simulink subsystem "DiscreteTimeController"  (R2020b)
settings: Solver=VariableStepAuto  StartTime=0.0  StopTime=10.0  RelTol=1e-3
model mask{Ts=-1, forward_action_enabled=0, use_lambda_const=on, lambdaT_const=0, use_max_analytic_lambda=on, rmse_noise_level=0, l_fcn_disabled=on, val_min=[], rmse_noise_slope_max=[], rmse_noise_min=[]}
settings Model: Creator=marco  LastModifiedBy=marco

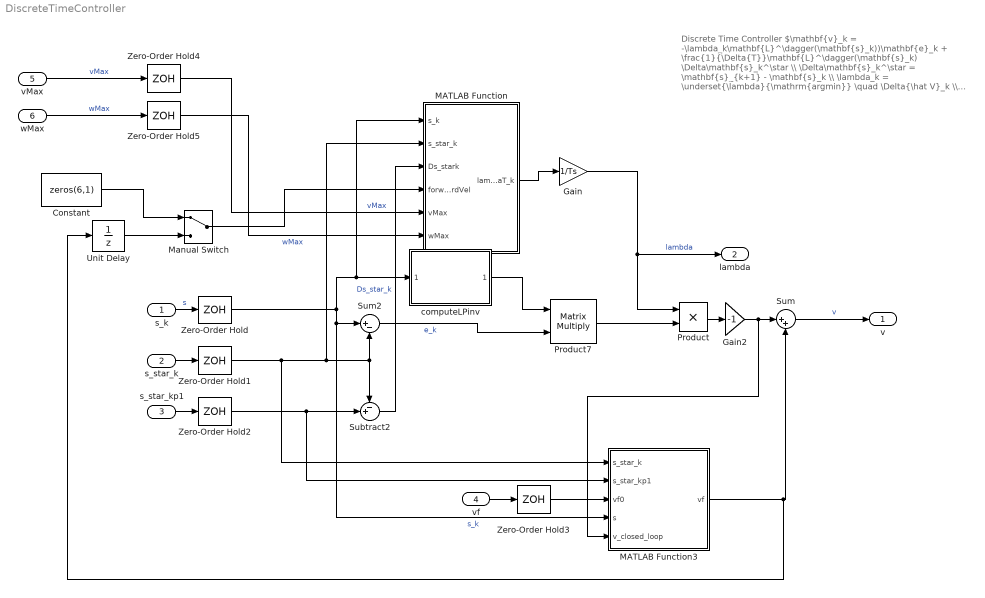
== system DiscreteTimeController ==
  note: Discrete Time Controller
      | $\mathbf{v}_k = -\lambda_k\mathbf{L}^\dagger(\mathbf{s}_k))\mathbf{e}_k + \frac{1}{\Delta{T}}\mathbf{L}^\dagger(\mathbf{s}_k) \Delta\mathbf{s}_k^\star \\ \Delta\mathbf{s}_k^\star = \mathbf{s}_{k+1} - \mathbf{s}_k \\ \lambda_k = \underset{\lambda}{\mathrm{argmin}} \quad \Delta{\hat V}_k \\ \textrm{s.t.} \quad \textrm{velocity limits}$
  s_k : Inport
  s_star_k : Inport  Port=2
  s_star_kp1 : Inport  Port=3
  vf : Inport  Port=4
  vMax : Inport  Port=5
  wMax : Inport  Port=6
  Constant : Constant  Value=zeros(6,1)
  Gain : Gain  Gain=1/Ts
  Gain2 : Gain  Gain=-1
  MATLAB Function : MATLAB Function  TreatAsAtomicUnit=on
  MATLAB Function3 : MATLAB Function  TreatAsAtomicUnit=on
  Manual Switch : ManualSwitch
  Product : Product
  Product7 : Product  Multiplication=Matrix(*)
  Subtract2 : Sum  Inputs=-+|
  Sum : Sum  Inputs=|++
  Sum2 : Sum  Inputs=|+-
  Unit Delay : UnitDelay  SampleTime=Ts  HasFrameUpgradeWarning=on
  Zero-Order Hold{,1..5} (6 alike) : ZeroOrderHold  SampleTime=Ts
  computeLPinv : Subsystem  ReferencedSubsystem=computeLPinv
  v : Outport
  lambda : Outport  Port=2
  wires:
  vf/1 -> Zero-Order Hold3/1
  Product/1 -> Gain2/1
  MATLAB Function3/1(vf) -> Sum/2, Unit Delay/1
  s_star_kp1/1 -> Zero-Order Hold2/1
  computeLPinv/1 -> Product7/1
  Sum/1 -> v/1  "v"
  Gain2/1 -> Sum/1, MATLAB Function3/5(v_closed_loop)
  Gain/1 -> Product/1, lambda/1  "lambda"
  Product7/1 -> Product/2
  s_star_k/1 -> Zero-Order Hold1/1
  s_k/1 -> Zero-Order Hold/1  "s"
  Subtract2/1 -> MATLAB Function/3(Ds_stark)  "Ds_star_k"
  Zero-Order Hold/1 -> computeLPinv/1, MATLAB Function/1(s_k), Sum2/1, MATLAB Function3/4(s)  "s_k"
  MATLAB Function/1(lambdaT_k) -> Gain/1
  Zero-Order Hold1/1 -> MATLAB Function3/1(s_star_k), Subtract2/1, Sum2/2, MATLAB Function/2(s_star_k)
  Zero-Order Hold2/1 -> Subtract2/2, MATLAB Function3/2(s_star_kp1)
  Zero-Order Hold3/1 -> MATLAB Function3/3(vf0)
  Sum2/1 -> Product7/2  "e_k"
  Manual Switch/1 -> MATLAB Function/4(forwardVel)
  Constant/1 -> Manual Switch/1
  Unit Delay/1 -> Manual Switch/2
  wMax/1 -> Zero-Order Hold5/1  "wMax"
  vMax/1 -> Zero-Order Hold4/1  "vMax"
  Zero-Order Hold4/1 -> MATLAB Function/5(vMax)  "vMax"
  Zero-Order Hold5/1 -> MATLAB Function/6(wMax)  "wMax"

== matlab function DiscreteTimeController/MATLAB Function ==
  data: s_k input; lambdaT_k output; s_star_k input; Ds_stark input; Ts parameter double; use_lambda_const parameter boolean; lambdaT_const parameter double; use_max_analytic_lambda parameter boolean; rmse_noise_level parameter; forwardVel input boolean; rmse_noise_min parameter; rmse_noise_slope_max parameter; val_min parameter; vMax input double; wMax input double; l_fcn_disabled parameter
function lambdaT_k  = fcn(s_k, s_star_k, Ds_stark, Ts, use_lambda_const, lambdaT_const, use_max_analytic_lambda, rmse_noise_level, forwardVel, rmse_noise_min, rmse_noise_slope_max, val_min, vMax, wMax,l_fcn_disabled)
coder.extrinsic('opt_problem_lambdaT'); % <- Informing the Coder

TForwardVel = Ts*forwardVel(:);
TForwardVel = []; % in the paper the controller does not consider directly the presence of a forward vel
                  % it works but it is not in the proofs

       
l_fcn = @(rmse)linear_l_fcn(rmse, rmse_noise_min, rmse_noise_slope_max, val_min, l_fcn_disabled);

if use_lambda_const
    lambdaT_k = lambdaT_const;
    return;
end

ek = s_k-s_star_k;

analitic_lambdaT_max = ...
    computeAnaliticLambdaTMax( ...
       ek, ...
       computeL(s_k), ...
       Ds_stark, ...
       TForwardVel, ...
       rmse_noise_level, ...
       l_fcn ...
       );

if use_max_analytic_lambda
    lambdaT_k = analiticLambdaTWithVelLimits( ...
        analitic_lambdaT_max, ...
        ek, ...
        s_star_k, ...
        vMax*Ts, ...
        wMax*Ts, ...
        TForwardVel ...
        );
   return;
end

lambdaT_k = opt_problem_lambdaT(...
    ek, ...
    s_star_k, ...
    vMax*Ts, ...
    wMax*Ts, ...
    Ds_stark, ...
    TForwardVel, ...
    rmse_noise_level, ...
    analitic_lambdaT_max ...
    );

== matlab function DiscreteTimeController/MATLAB Function3 ==
  data: s_star_k input; vf output; s_star_kp1 input; vf0 input; s input; v_closed_loop input; Ts parameter; forward_action_enabled parameter
function vf  = sim_forw_action(s_star_k,s_star_kp1, vf0, s, v_closed_loop,  Ts, forward_action_enabled)
    if forward_action_enabled
%         vf0 = zeros(6,1);
        vf = computeForwardAction(s_star_k, s_star_kp1, Ts, vf0, s, v_closed_loop(4:6));
    else
        vf = zeros(6,1);
%         vf = computeForwardAction(s_star_k, s_star_k, Ts, vf0);
    end
